simulink library "calcThrDrag_ul"  (R2020a)
settings: Solver=VariableStepAuto  StartTime=0.0  StopTime=10.0  RelTol=1e-3
libraries: vrlib x1
settings Model: Creator=Ayaz  LastModifiedBy=Ayaz

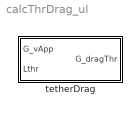
== system calcThrDrag_ul ==
  tetherDrag : Subsystem  mask{dThr=0, CdThr=0, rhoAir=0}
      mask prompts: dThr "Tether diameter [m]"; CdThr "Tether drag coefficient [-]"; rhoAir "Air density [kg/m^3]"

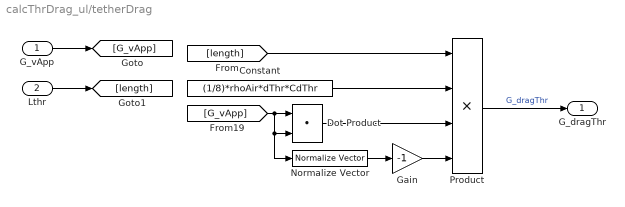
== system calcThrDrag_ul/tetherDrag ==
  G_vApp : Inport
  Lthr : Inport  Port=2
  Constant : Constant  Value=(1/8)*rhoAir*dThr*CdThr
  Dot Product : DotProduct  InputSameDT=on  OutDataTypeStr=Inherit: Inherit via internal rule
  Gain : Gain  Gain=-1
  Normalize Vector : vrlib/Utilities/Normalize Vector  maxzero=0
  Product : Product  Inputs=4
  G_dragThr : Outport
  wires:
  G_vApp/1 -> [G_vApp]
  Lthr/1 -> [length]
  [G_vApp] -> Normalize Vector/1, Dot Product/2, Dot Product/1
  [length] -> Product/1
  Constant/1 -> Product/2
  Dot Product/1 -> Product/3
  Normalize Vector/1 -> Gain/1
  Product/1 -> G_dragThr/1  "G_dragThr"
  Gain/1 -> Product/4
